simulink subsystem "DiagnosticManagement"  (R2019b)
settings: Solver=VariableStepAuto  StartTime=0.0  StopTime=10.0  RelTol=1e-3
undefined symbols (not defined in the file): __PRM__SERIALIZED__DATA__, SubsystemReferenceBlock
libraries: FunctionCallDivider x2
settings Model: Creator=Nick  LastModifiedBy=Nick

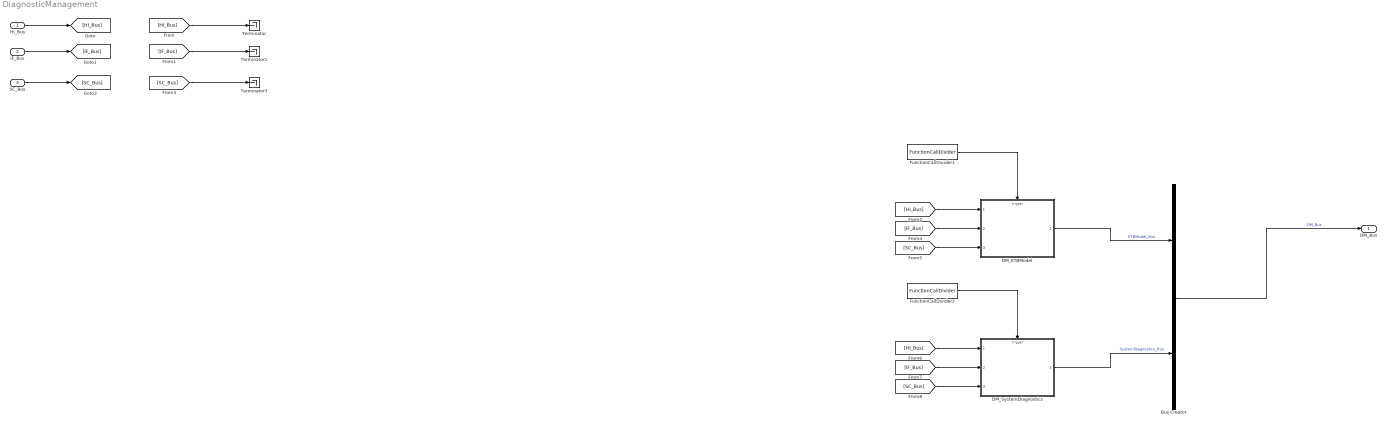
== system DiagnosticManagement ==
  HI_Bus : Inport
  IF_Bus : Inport  Port=2
  SC_Bus : Inport  Port=3
  Bus Creator : BusCreator  Inputs=2
  DM_ETBModel : Subsystem  BlockKeywords=__PRM__SERIALIZED__DATA__:SubsystemReferenceBlock  ReferencedSubsystem=DM_ETBModel
  DM_SystemDiagnostics : Subsystem  BlockKeywords=__PRM__SERIALIZED__DATA__:SubsystemReferenceBlock  ReferencedSubsystem=DM_SystemDiagnostics
  FunctionCallDivider1 : FunctionCallDivider/Algroithms/FunctionCallDivider  counts=1
  FunctionCallDivider2 : FunctionCallDivider/Algroithms/FunctionCallDivider  counts=10
  Terminator : Terminator
  Terminator1 : Terminator
  Terminator3 : Terminator
  DM_Bus : Outport
  wires:
  [HI_Bus] -> Terminator/1
  [IF_Bus] -> Terminator1/1
  HI_Bus/1 -> [HI_Bus]
  IF_Bus/1 -> [IF_Bus]
  Bus Creator/1 -> DM_Bus/1  "DM_Bus"
  [SC_Bus] -> Terminator3/1
  SC_Bus/1 -> [SC_Bus]
  FunctionCallDivider1/1 -> DM_ETBModel/Trigger
  [HI_Bus] -> DM_ETBModel/1
  [IF_Bus] -> DM_ETBModel/2
  [SC_Bus] -> DM_ETBModel/3
  DM_ETBModel/1 -> Bus Creator/1  "ETBModel_Bus"
  FunctionCallDivider2/1 -> DM_SystemDiagnostics/Trigger
  [IF_Bus] -> DM_SystemDiagnostics/2
  [HI_Bus] -> DM_SystemDiagnostics/1
  [SC_Bus] -> DM_SystemDiagnostics/3
  DM_SystemDiagnostics/1 -> Bus Creator/2  "SystemDiagnostics_Bus"
